simulink model "hall_effect"  (R2024b)
settings: Solver=FixedStepAuto  StartTime=0.0  StopTime=inf  RelTol=1e-3  EnableMultiTasking=on
libraries: stm32f4xxblockslib x2, simulink x1
settings Model: STM32="{\"AnalogInput\":[{\"ID\":\"untitled:1\"},{\"ID\":\"Poten:1\"},{\"ID\":\"hall_effect:1\"}],\"DigitalPortRead\":[{\"ID\":\"untitled:21\"},{\"ID\":\"Poten:21\"},{\"ID\":\"hall_effect:21\"}]}"  Creator=rew1m  LastModifiedBy=janej
settings OptimizationCC: DefaultParameterBehavior=Inlined  EnhancedBackFolding=on  PassReuseOutputArgsAs=Individual arguments  ZeroExternalMemoryAtStartup=off  ZeroInternalMemoryAtStartup=off  MaxStackSize=512  OptimizeBlockOrder=speed  DifferentSizesBufferReuse=on  OptimizationCustomize=off  EfficientTunableParamExpr=on
settings DebuggingCC: ParameterTunabilityLossMsg=error
settings HardwareCC: ProdBitPerPointer=32  ProdBitPerSizeT=32  ProdBitPerPtrDiffT=32  ProdLargestAtomicInteger=Long  ProdLargestAtomicFloat=Double  ProdWordSize=32  ProdLongLongMode=on  ProdHWDeviceType=ARM Compatible->ARM Cortex-M
settings SFSimCC: MATLABDynamicMemAlloc=off
settings RTWCC: Description=Embedded Coder  SystemTargetFile=ert.tlc  HardwareBoard=STM32G4xx Based  TemplateMakefile=ert_default_tmf  Toolchain=GNU Tools for ARM Embedded Processors
settings CodeAppCC: ForceParamTrailComments=on  IgnoreCustomStorageClasses=off  OperatorAnnotations=on  SimulinkDataObjDesc=on  SFDataObjDesc=on  InsertBlockDesc=on
settings ERTTargetCC: TargetLangStandard=C99 (ISO)  CodeReplacementLibrary=ARM Cortex-M  ExtModeTransport=3  ExtModeStaticAlloc=on  ExtModeStaticAllocSize=2048  ExtModeMexFile=ext_xcp  ExtModeIntrfLevel=Level2 - Open

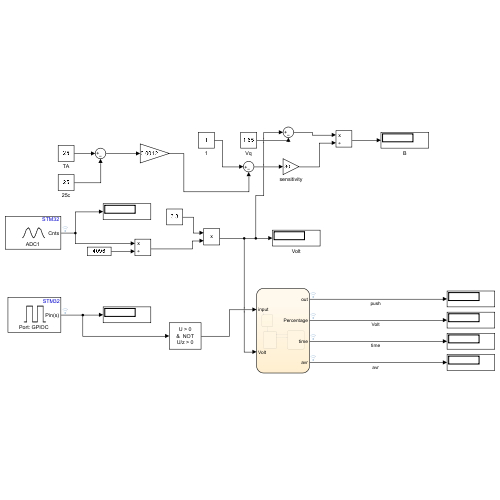
[thumbnail: Simulink's stored preview of the top-level diagram]
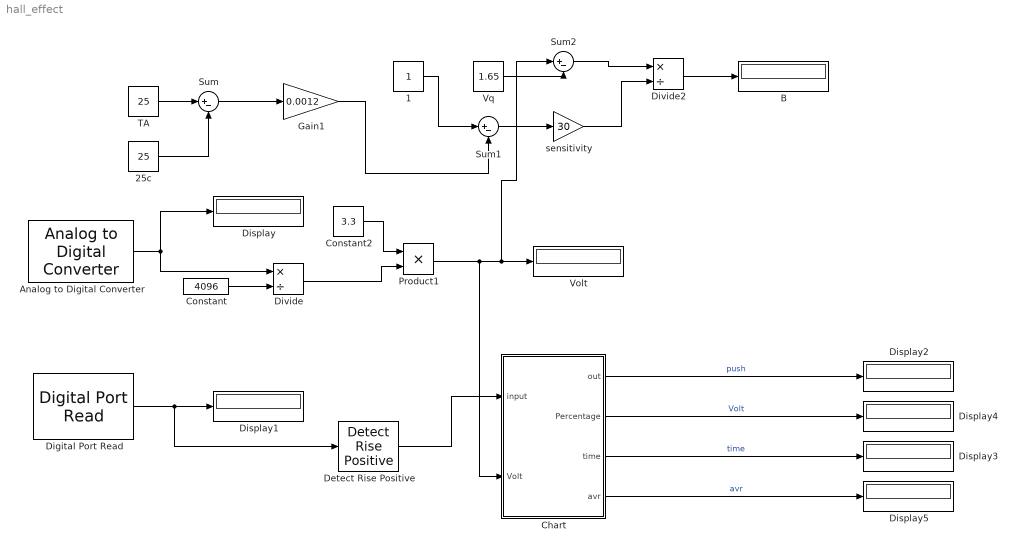
== system hall_effect ==
  1 : Constant
  25c : Constant  Value=25
  Analog to Digital Converter : stm32f4xxblockslib/Analog to Digital Converter  ADCModule=ADC1  ConversionGroup=Regular  TriggerMode=Trigger and read  NumberOfConversions=1  EnableBufferConv=off  BufferLength=1  OutputStatus=off  SampleTime=-1  EnableSimPort=off  hoistedMaskSrc=ECSoC/ECSimCodegen/Analog to Digital Converter
  B : Display
  Chart : Stateflow chart  TreatAsAtomicUnit=on
  Constant : Constant  Value=4096
  Constant2 : Constant  Value=3.3
  Detect Rise Positive : simulink/Logic and Bit Operations/Detect Rise Positive  vinit=0  OutDataTypeStr=boolean
  Digital Port Read : stm32f4xxblockslib/Digital Port Read  PortName=GPIOC  PinNumber=[13]  ReadOperation=on  IOAsArray=on  SampleTime=-1  EnableSimPort=off  hoistedMaskSrc=ECSoC/ECSimCodegen/Digital Port Read
  Display{,1..5} (6 alike) : Display
  Divide : Product  Inputs=*/
  Divide2 : Product  Inputs=*/
  Gain1 : Gain  Gain=0.0012
  Product1 : Product
  Sum : Sum  Inputs=|+-
  Sum1 : Sum  Inputs=|+-
  Sum2 : Sum  Inputs=|+-
  TA : Constant  Value=25
  Volt : Display
  Vq : Constant  Value=1.65
  sensitivity : Gain  Gain=30
  wires:
  Analog to Digital Converter/1 -> Display/1, Divide/1
  Constant/1 -> Divide/2
  Divide/1 -> Product1/2
  Constant2/1 -> Product1/1
  Product1/1 -> Volt/1, Sum2/1, Chart/2(Volt)
  Digital Port Read/1 -> Detect Rise Positive/1, Display1/1
  Detect Rise Positive/1 -> Chart/1(input)
  Chart/1(out) -> Display2/1  "push"
  Chart/3(time) -> Display3/1  "time"
  Chart/2(Percentage) -> Display4/1  "Volt"
  Chart/4(avr) -> Display5/1  "avr"
  TA/1 -> Sum/1
  25c/1 -> Sum/2
  Gain1/1 -> Sum1/2
  Sum/1 -> Gain1/1
  1/1 -> Sum1/1
  Sum1/1 -> sensitivity/1
  Vq/1 -> Sum2/2
  Sum2/1 -> Divide2/1
  sensitivity/1 -> Divide2/2
  Divide2/1 -> B/1

== stateflow chart hall_effect/Chart ==
  state Inital
    time = 0;
    out = 0;
    total = 0;
    avr = 0;
    round = 1;
  state HIGHT
    entry:
    out = 1;
    time = 0.01;
    avr = 0;
    during:
    time = time + 0.002
    Volt = Volt
    total = total + Volt
    round = round + 1
  state Low
    entry:
    out = 0;
    avr = total/round
    total = 0;
    round = 0;
  (default) -> Inital
  Inital -> Low
  HIGHT -> Low : [round >= 1000]
  Low -> HIGHT : [input == 1]
  data: out output; Percentage output; input input; time output; Volt input; avr output; total local; round local
